simulink model "PID_Control"  (R2025b)
settings: Solver=VariableStepAuto  StartTime=0.0  StopTime=10  RelTol=1e-3
values from neighbouring files (symbols this model uses):
  B = 1    [PID_Control_Script.m]
  d = 0.8    [PID_Control_Script.m]
  J = 3    [PID_Control_Script.m]
  Kd = 2*(zeta*wn*J) - B    (= 11)    [PID_Control_Script.m]
  Ki = 4.8    [PID_Control_Script.m]
  Kp = (J * wn^2)    (= 12)    [PID_Control_Script.m]
libraries: simulink_extras x1
settings Model: Creator=Yami  LastModifiedBy=Yami

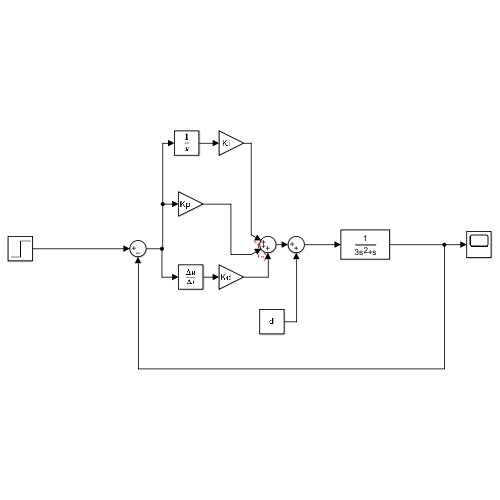
[thumbnail: Simulink's stored preview of the top-level diagram]
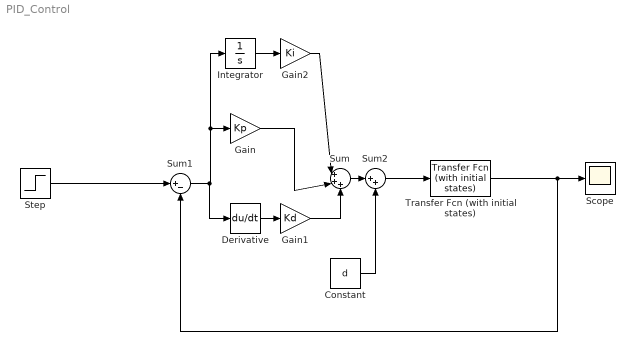
== system PID_Control ==
  Constant : Constant  Value=d
  Derivative : Derivative
  Gain : Gain  Gain=Kp
  Gain1 : Gain  Gain=Kd
  Gain2 : Gain  Gain=Ki
  Integrator : Integrator
  Scope : Scope
      settings: ActiveDisplayYMinimum=-0.12499908340341713  ActiveDisplayYMaximum=1.1249917506307545
  Step : Step  SampleTime=0
  Sum : Sum  Inputs=|+++
  Sum1 : Sum  Inputs=|+-
  Sum2 : Sum  Inputs=|++
  Transfer Fcn (with initial states) : simulink_extras/Additional Linear/Transfer Fcn (with initial states)  N=[1]  D=[J B 0]  X0=0
  wires:
  Step/1 -> Sum1/1
  Transfer Fcn (with initial states)/1 -> Sum1/2, Scope/1
  Sum1/1 -> Derivative/1, Integrator/1, Gain/1
  Derivative/1 -> Gain1/1
  Constant/1 -> Sum2/2
  Sum2/1 -> Transfer Fcn (with initial states)/1
  Integrator/1 -> Gain2/1
  Sum/1 -> Sum2/1
  ? -> ?
  Gain1/1 -> Sum/3
  Gain/1 -> Sum/2
  Gain2/1 -> Sum/1
